simulink model "Assignment3Sim"  (R2020b)
settings: Solver=VariableStepAuto  StartTime=0.0  StopTime=86400  RelTol=1e-3
values from neighbouring files (symbols this model uses):
  freq1 = 100    [Assignment3Mat.m]
  freq2 = 1    [Assignment3Mat.m]
  k1 = 2    [Assignment3Mat.m]
  noiseAmp = 0.001    [Assignment3Mat.m]
  noiseFreq = 50    [Assignment3Mat.m]
settings Model: Creator=Paolo  LastModifiedBy=Paolo

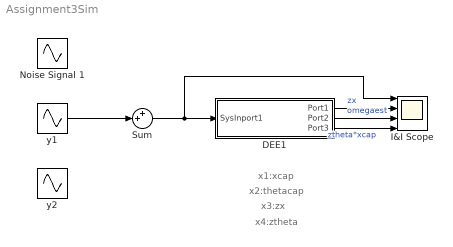
== system Assignment3Sim ==
  note: x4:ztheta
  note: x3:zx
  note: x2:thetacap
  note: x1:xcap
  DEE1 : Subsystem  mask(Differential Equation Editor (DEE)){}
      settings: OpenFcn=diffeqed
      mask Display: disp('Stimatore I&I')
  I&I Scope : Scope  NumInputPorts=4
  Noise Signal 1 : Sin  Amplitude=noiseAmp  Frequency=noiseFreq  SampleTime=0
  Sum : Sum  Inputs=++|
  y1 : Sin  Frequency=freq1  SampleTime=0
  y2 : Sin  Frequency=freq2  SampleTime=0
  wires:
  Sum/1 -> I&I Scope/1, DEE1/1(SysInport1)
  DEE1/3(Port3) -> I&I Scope/4  "ztheta*xcap"
  DEE1/1(Port1) -> I&I Scope/2  "zx"
  DEE1/2(Port2) -> I&I Scope/3  "omegaest"
  y1/1 -> Sum/2

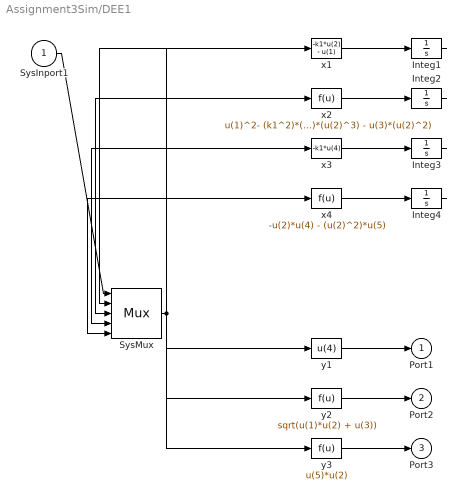
== system Assignment3Sim/DEE1 ==
  SysInport1 : Inport
  Integ1 : Integrator
  Integ2 : Integrator
  Integ3 : Integrator  InitialCondition=1
  Integ4 : Integrator  InitialCondition=1
  SysMux : Mux  Inputs=5
  x1 : Fcn  Expr=-k1*u(2) - u(1)
  x2 : Fcn  Expr=u(1)^2- (k1^2)*(u(2)^2) - u(1)*(u(2)^3) - u(3)*(u(2)^2)
  x3 : Fcn  Expr=-k1*u(4)
  x4 : Fcn  Expr=-u(2)*u(4) - (u(2)^2)*u(5)
  y1 : Fcn  Expr=u(4)
  y2 : Fcn  Expr=sqrt(u(1)*u(2) + u(3))
  y3 : Fcn  Expr=u(5)*u(2)
  Port1 : Outport
  Port2 : Outport  Port=2
  Port3 : Outport  Port=3
  wires:
  SysInport1/1 -> SysMux/1
  SysMux/1 -> x1/1, x2/1, x3/1, x4/1, y1/1, y2/1, y3/1
  x1/1 -> Integ1/1
  Integ1/1 -> SysMux/2
  x2/1 -> Integ2/1
  Integ2/1 -> SysMux/3
  x3/1 -> Integ3/1
  Integ3/1 -> SysMux/4
  x4/1 -> Integ4/1
  Integ4/1 -> SysMux/5
  y1/1 -> Port1/1
  y2/1 -> Port2/1
  y3/1 -> Port3/1
